simulink model "drone_control_definitivo"  (R2018a)
settings: Solver=FixedStepAuto  StartTime=0.0  StopTime=inf  FixedStep=sample_time  RelTol=1e-3
PostLoadFcn:
  | load('drone_buses.mat');
model workspace (MAT data in the model file):
  SL_ROS_VariableLengthArrays_MaxSizes.CommonInfo.ArrayTruncateAction = 'EmitWarning'
  SL_ROS_VariableLengthArrays_MaxSizes.MsgTypeMap = containers.Map
  SL_ROS_VariableLengthArrays_MaxSizes.MsgTypeMap.serialization.keys = {'sensor_msgs/Image'}
  SL_ROS_VariableLengthArrays_MaxSizes.MsgTypeMap.serialization.values{1}(1).PropertyName = 'Data'
  SL_ROS_VariableLengthArrays_MaxSizes.MsgTypeMap.serialization.values{1}(1).DataType = 'uint8'
  SL_ROS_VariableLengthArrays_MaxSizes.MsgTypeMap.serialization.values{1}(1).MaxLength = 230400
  SL_ROS_VariableLengthArrays_MaxSizes.MsgTypeMap.serialization.values{1}(2).PropertyName = 'Encoding'
  SL_ROS_VariableLengthArrays_MaxSizes.MsgTypeMap.serialization.values{1}(2).DataType = 'uint8'
  SL_ROS_VariableLengthArrays_MaxSizes.MsgTypeMap.serialization.values{1}(2).MaxLength = 128
  SL_ROS_VariableLengthArrays_MaxSizes.MsgTypeMap.serialization.uniformity = 0
  SL_ROS_VariableLengthArrays_MaxSizes.MsgTypeMap.serialization.keyType = 'char'
  SL_ROS_VariableLengthArrays_MaxSizes.MsgTypeMap.serialization.valueType = 'any'
  cmd_calibration = 0.4
  sample_time = 0.05
undefined symbols (not defined in the file or in its folder): Orientation, Position
libraries: robotlib x4, simulink_extras x2, simulink x2, aerolibanimutils x1
settings Model: Creator=rcasado  LastModifiedBy=dronechallenge
settings OptimizationCC: EnhancedBackFolding=on  PassReuseOutputArgsAs=Individual arguments  MaxStackSize=64  OptimizeBlockOrder=speed  DifferentSizesBufferReuse=on  OptimizationCustomize=off
settings DebuggingCC: ParameterTunabilityLossMsg=error  BusObjectLabelMismatch=none
settings HardwareCC: ProdBitPerPointer=32  ProdBitPerSizeT=32  ProdBitPerPtrDiffT=32  ProdLargestAtomicFloat=None  ProdIntDivRoundTo=Undefined  ProdEndianess=Unspecified  ProdWordSize=32  ProdHWDeviceType=Generic->Unspecified (assume 32-bit Generic)
settings SFSimCC: MATLABDynamicMemAlloc=off
settings RTWCC: SystemTargetFile=ert.tlc  HardwareBoard=Robot Operating System (ROS)  TLCOptions="-aInlineSetEventsForThisBaseRateFcn=TLC_FALSE -aSuppressMultiTaskScheduler=TLC_FALSE  -aRateBasedStepFcn=0"  TemplateMakefile=ert_default_tmf  GenerateReport=on  Toolchain=Catkin  IncludeHyperlinkInReport=on  LaunchReport=on  TargetLang=C++  GenerateTraceInfo=on  GenerateTraceReport=on  GenerateTraceReportSl=on  GenerateTraceReportSf=on  GenerateTraceReportEml=on
settings CodeAppCC: ForceParamTrailComments=on  IgnoreCustomStorageClasses=off  OperatorAnnotations=on  SimulinkDataObjDesc=on  SFDataObjDesc=on  InsertBlockDesc=on

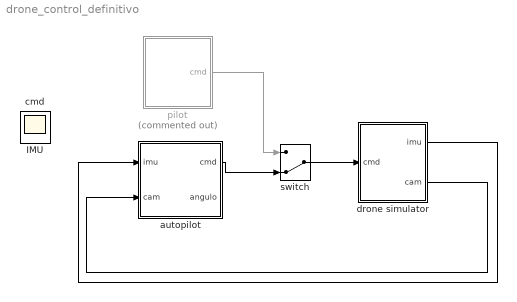
== system drone_control_definitivo ==
  autopilot : Stateflow chart  TreatAsAtomicUnit=on
  drone simulator : Subsystem
      mask Display:
      | patch([50 -50 -50 50], [40 40 -60 -60], [1 1 1])
      | 
      | patch([8 -8 -8 8], [6 6 -6 -6], [0.7 0.7 0.7])
      | 
      | patch([ 8  8  28  28], [2 0 0 2], [0.5 0.5 0.5])
      | patch([-8 -8 -28 -28], [2 0 0 2], [0.5 0.5 0.5])
      | 
      | patch([ 30  46  30  14], [6 5 4 5], [1 1 0])
      | patch([-30 -46 -30 -14], [6 5 4 5], [1 1 0])
      | 
      | patch([ 28  28  32  32], [4 -2 -2 4], [0 0 0])
      | patch([-28 -28 -32 -32], [4 -2 -2 4], [0 0 0])
      | 
      | patch([ 8  12  11  7], [-6 -18 -18 -6], [0 0 0])
      | patch([-8 -12 -11 -7], [-6 -18 -18 -6], [0 0 0])
  pilot : Subsystem  Commented=on
      mask Display:
      | patch([12 -2 -2 12], [12 12 -2 -2], [0.9 0.9 0.9])
      | 
      | % bola roja
      | patch([4 6 7 7 6 4 3 3], [6 6 7 9 10 10 9 7], [1 0 0])
      | 
      | % palo gris
      | patch([4 6 6 4], [3 3 6 6], [0.2 0.2 0.2])
      | 
      | % base negra
      | patch([1 9 10 10 9 1 0 0], [0 0 1 2 3 3 2 1], [0 0 0])
  switch : ManualSwitch  CurrentSetting=0
  IMU : Scope
  cmd : Scope
  wires:
  pilot/1(cmd) -> switch/1
  switch/1 -> drone simulator/1(cmd)
  autopilot/1(cmd) -> switch/2
  drone simulator/1(imu) -> autopilot/1(imu)
  drone simulator/2(cam) -> autopilot/2(cam)

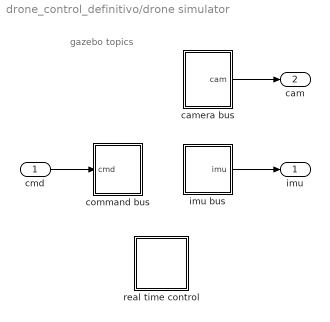
== system drone_control_definitivo/drone simulator ==
  note: gazebo
      | topics
  cmd : Inport
  camera bus : Subsystem
  command bus : Subsystem
  imu bus : Subsystem
  real time control : Subsystem
      mask Display: disp('realtime\ncontrol')
  imu : Outport
  cam : Outport  Port=2
  wires:
  imu bus/1(imu) -> imu/1
  cmd/1 -> command bus/1(cmd)
  camera bus/1(cam) -> cam/1

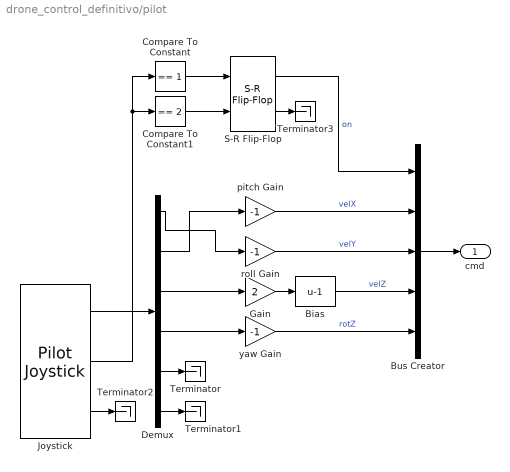
== system drone_control_definitivo/pilot ==
  Bias : Bias  Bias=-1
  Bus Creator : BusCreator  Inputs=5  OutDataTypeStr=Bus: bus_command  NonVirtualBus=on
      settings: InheritFromInputs=off
  Compare To Constant : simulink/Logic and Bit Operations/Compare To Constant  relop===  const=1  OutDataTypeStr=boolean
  Compare To Constant1 : simulink/Logic and Bit Operations/Compare To Constant  relop===  const=2  OutDataTypeStr=boolean
  Demux : Demux  Outputs=6
  Gain : Gain  Gain=2
  Joystick : aerolibanimutils/Pilot Joystick  JoystickID=Joystick1  OutputConfiguration=AllOutputs  SampleTime=sample_time
  S-R Flip-Flop : simulink_extras/Flip Flops/S-R Flip-Flop  initial_condition=0
  Terminator{,1..3} (4 alike) : Terminator
  pitch Gain : Gain  Gain=-1
  roll Gain : Gain  Gain=-1
  yaw Gain : Gain  Gain=-1
  cmd : Outport
  wires:
  Demux/4 -> yaw Gain/1
  Demux/3 -> Gain/1
  Demux/1 -> roll Gain/1
  Demux/2 -> pitch Gain/1
  Gain/1 -> Bias/1
  Bias/1 -> Bus Creator/4  "velZ"
  yaw Gain/1 -> Bus Creator/5  "rotZ"
  pitch Gain/1 -> Bus Creator/2  "velX"
  roll Gain/1 -> Bus Creator/3  "velY"
  S-R Flip-Flop/1 -> Bus Creator/1  "on"
  Bus Creator/1 -> cmd/1
  Joystick/1 -> Demux/1
  Demux/6 -> Terminator1/1
  Demux/5 -> Terminator/1
  Joystick/2 -> Compare To Constant/1, Compare To Constant1/1
  Joystick/3 -> Terminator2/1
  Compare To Constant/1 -> S-R Flip-Flop/1
  Compare To Constant1/1 -> S-R Flip-Flop/2
  S-R Flip-Flop/2 -> Terminator3/1

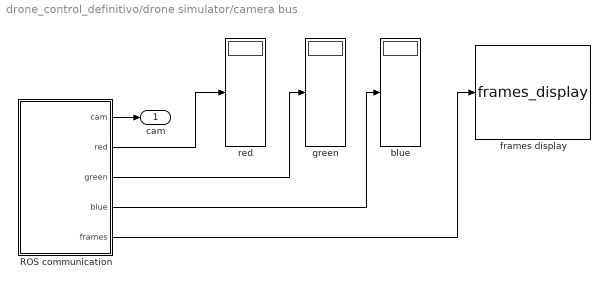
== system drone_control_definitivo/drone simulator/camera bus ==
  ROS communication : Subsystem
  blue : Display
  frames display : MATLABFcn  StartFcn=|  MATLABFcn=frames_display  OutputDimensions=0  Output1D=off
      | clear functions;
      | clc;
      mask Display:
      | patch([80 100 100 80], [60 60 80 80],[1 0 0])
      | 
      | patch([60 75 75 60], [20 20 30 30],[0 1 0])
      | 
      | patch([20 40 40 20], [40 40 50 50],[0 0 1])
  green : Display
  red : Display
  cam : Outport
  wires:
  ROS communication/2(red) -> red/1
  ROS communication/3(green) -> green/1
  ROS communication/4(blue) -> blue/1
  ROS communication/1(cam) -> cam/1
  ROS communication/5(frames) -> frames display/1

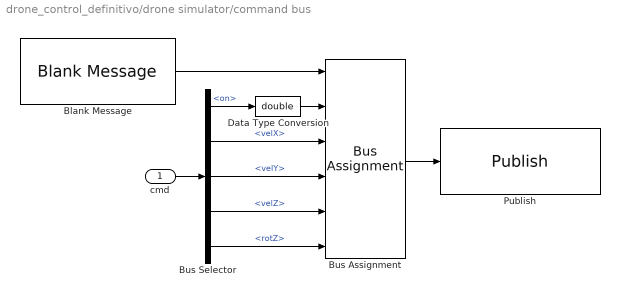
== system drone_control_definitivo/drone simulator/command bus ==
  cmd : Inport
  Blank Message : robotlib/Blank Message  SourceLibraryInfo=This block requires Robotics System Toolbox  messageType=geometry_msgs/Pose  SampleTime=sample_time
      settings: SourceProductBaseCode=RO
  Bus Assignment : BusAssignment  AssignedSignals=Position.X,Orientation.X,Orientation.Y,Orientation.Z,Orientation.W
  Bus Selector : BusSelector  OutputSignals=on,velX,velY,velZ,rotZ
  Data Type Conversion : DataTypeConversion  OutDataTypeStr=double
  Publish : robotlib/Publish  SourceLibraryInfo=This block requires Robotics System Toolbox  topicSource=Select from ROS network  topic=/quadcopter/bus_command  messageType=geometry_msgs/Pose  messageQueueLength=105
      settings: SourceProductBaseCode=RO
  wires:
  Bus Assignment/1 -> Publish/1
  cmd/1 -> Bus Selector/1
  Blank Message/1 -> Bus Assignment/1
  Bus Selector/4 -> Bus Assignment/5  "<velZ>"
  Bus Selector/3 -> Bus Assignment/4  "<velY>"
  Bus Selector/2 -> Bus Assignment/3  "<velX>"
  Bus Selector/1 -> Data Type Conversion/1  "<on>"
  Bus Selector/5 -> Bus Assignment/6  "<rotZ>"
  Data Type Conversion/1 -> Bus Assignment/2

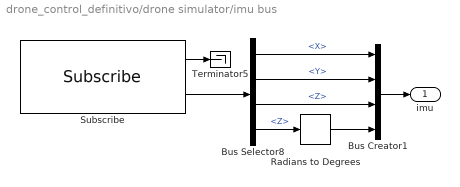
== system drone_control_definitivo/drone simulator/imu bus ==
  Bus Creator1 : BusCreator  Inputs=4  OutDataTypeStr=Bus: bus_IMU  NonVirtualBus=on
      settings: InheritFromInputs=off
  Bus Selector8 : BusSelector  DialogController=Simulink.DDGSource_BusSelector  OutputSignals=Pose.Position.X,Pose.Position.Y,Pose.Position.Z,Pose.Orientation.Z
  Radians to Degrees : simulink_extras/Transformations/Radians to Degrees
  Subscribe : robotlib/Subscribe  SourceLibraryInfo=This block requires Robotics System Toolbox  topicSource=Select from ROS network  topic=/quadcopter/odometry  messageType=gazebo_msgs/ModelState  sampleTime=sample_time  messageQueueLength=51
      settings: SourceProductBaseCode=RO
  Terminator5 : Terminator
  imu : Outport
  wires:
  Subscribe/1 -> Terminator5/1
  Bus Selector8/4 -> Radians to Degrees/1  "<Z>"
  Bus Selector8/2 -> Bus Creator1/2  "<Y>"
  Bus Selector8/3 -> Bus Creator1/3  "<Z>"
  Bus Selector8/1 -> Bus Creator1/1  "<X>"
  Bus Creator1/1 -> imu/1
  Radians to Degrees/1 -> Bus Creator1/4
  Subscribe/2 -> Bus Selector8/1

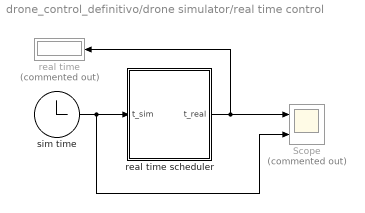
== system drone_control_definitivo/drone simulator/real time control ==
  Scope : Scope  Commented=on  NumInputPorts=2
  real time : Display  Commented=on
      settings: Format=bank
  real time scheduler : MATLAB Function  TreatAsAtomicUnit=on
  sim time : Clock
  wires:
  real time scheduler/1(t_real) -> real time/1, Scope/1
  sim time/1 -> real time scheduler/1(t_sim), Scope/2

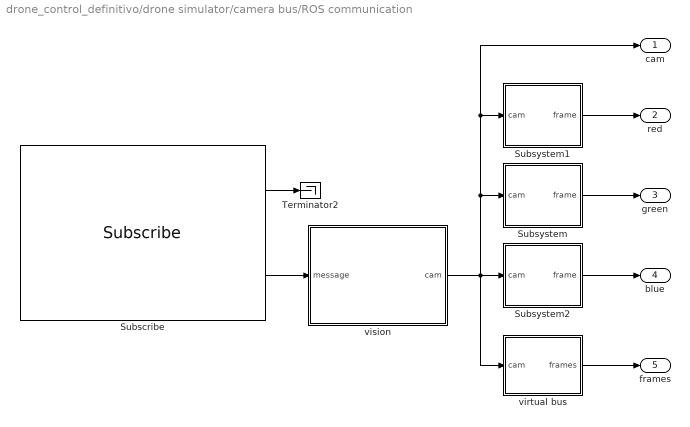
== system drone_control_definitivo/drone simulator/camera bus/ROS communication ==
  Subscribe : robotlib/Subscribe  SourceLibraryInfo=This block requires Robotics System Toolbox  topicSource=Select from ROS network  topic=/quadcopter/onboard_camera/image_raw  messageType=sensor_msgs/Image  sampleTime=sample_time  messageQueueLength=51
      settings: SourceProductBaseCode=RO
  Subsystem : Subsystem
  Subsystem1 : Subsystem
  Subsystem2 : Subsystem
  Terminator2 : Terminator
  virtual bus : Subsystem
  vision : MATLAB Function  TreatAsAtomicUnit=on
  cam : Outport
  red : Outport  Port=2
  green : Outport  Port=3
  blue : Outport  Port=4
  frames : Outport  Port=5
  wires:
  Subsystem/1(frame) -> green/1
  Subsystem1/1(frame) -> red/1
  Subsystem2/1(frame) -> blue/1
  virtual bus/1(frames) -> frames/1
  vision/1(cam) -> cam/1, Subsystem1/1(cam), Subsystem/1(cam), virtual bus/1(cam), Subsystem2/1(cam)
  Subscribe/2 -> vision/1(message)
  Subscribe/1 -> Terminator2/1

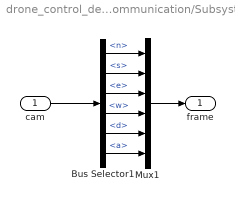
== system drone_control_definitivo/drone simulator/camera bus/ROS communication/Subsystem ==
  cam : Inport
  Bus Selector1 : BusSelector  OutputSignals=green.n,green.s,green.e,green.w,green.d,green.a
  Mux1 : Mux  Inputs=6
  frame : Outport
  wires:
  Bus Selector1/3 -> Mux1/3  "<e>"
  Bus Selector1/6 -> Mux1/6  "<a>"
  Bus Selector1/5 -> Mux1/5  "<d>"
  Bus Selector1/4 -> Mux1/4  "<w>"
  cam/1 -> Bus Selector1/1
  Bus Selector1/1 -> Mux1/1  "<n>"
  Mux1/1 -> frame/1
  Bus Selector1/2 -> Mux1/2  "<s>"

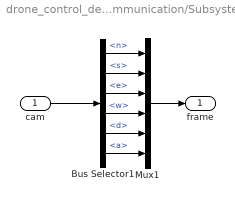
== system drone_control_definitivo/drone simulator/camera bus/ROS communication/Subsystem1 ==
  cam : Inport
  Bus Selector1 : BusSelector  OutputSignals=red.n,red.s,red.e,red.w,red.d,red.a
  Mux1 : Mux  Inputs=6
  frame : Outport
  wires:
  Bus Selector1/3 -> Mux1/3  "<e>"
  Bus Selector1/6 -> Mux1/6  "<a>"
  Bus Selector1/5 -> Mux1/5  "<d>"
  Bus Selector1/4 -> Mux1/4  "<w>"
  cam/1 -> Bus Selector1/1
  Bus Selector1/1 -> Mux1/1  "<n>"
  Mux1/1 -> frame/1
  Bus Selector1/2 -> Mux1/2  "<s>"

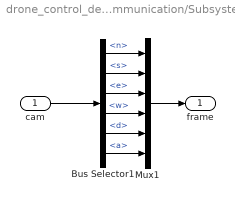
== system drone_control_definitivo/drone simulator/camera bus/ROS communication/Subsystem2 ==
  cam : Inport
  Bus Selector1 : BusSelector  OutputSignals=blue.n,blue.s,blue.e,blue.w,blue.d,blue.a
  Mux1 : Mux  Inputs=6
  frame : Outport
  wires:
  Bus Selector1/3 -> Mux1/3  "<e>"
  Bus Selector1/6 -> Mux1/6  "<a>"
  Bus Selector1/5 -> Mux1/5  "<d>"
  Bus Selector1/4 -> Mux1/4  "<w>"
  cam/1 -> Bus Selector1/1
  Bus Selector1/1 -> Mux1/1  "<n>"
  Mux1/1 -> frame/1
  Bus Selector1/2 -> Mux1/2  "<s>"

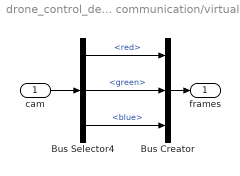
== system drone_control_definitivo/drone simulator/camera bus/ROS communication/virtual bus ==
  cam : Inport
  Bus Creator : BusCreator  Inputs=3  OutDataTypeStr=Bus: bus_camera
      settings: InheritFromInputs=off
  Bus Selector4 : BusSelector  OutputSignals=red,green,blue
  frames : Outport
  wires:
  Bus Selector4/1 -> Bus Creator/1  "<red>"
  Bus Selector4/3 -> Bus Creator/3  "<blue>"
  Bus Selector4/2 -> Bus Creator/2  "<green>"
  cam/1 -> Bus Selector4/1
  Bus Creator/1 -> frames/1

== matlab function drone_control_definitivo/drone simulator/real time control/real time scheduler ==
  data: t_sim input; t_real output
function t_real = fcn(t_sim)
%#codegen

coder.extrinsic('tic');
coder.extrinsic('toc');

persistent t0;
if isempty(t0)
    t0 = tic;
    t_real = 0;
end

t_real = toc(t0);

t_dif = t_sim - t_real;
if t_dif > 0
%    disp(t_dif)
    pause(t_dif);
end

t_real = toc(t0);
%disp(t_real)

== stateflow chart drone_control_definitivo/autopilot ==
  settings: updateMethod=DISCRETE  sampleTime=sample_time  executeAtInitialization=1
  state nav1 [parallel] [commented out]
    state inicio [commented out]
      entry:
      cmd.on=true;
    state AscenderA3m [commented out]
      entry:
      alturaFinal=3.00;
      during:
      velocidadZ=alturaFinal-imu.posZ;
      cmd.velZ=velocidadZ;
    state Suspendido [commented out]
      entry:
      cmd.velZ=0.00;
    state DescenderA2m [commented out]
      entry:
      alturaFinal=2.00;
      during:
      velocidadZ = alturaFinal-imu.posZ;
      cmd.velZ=velocidadZ;
    state Suspendido1 [commented out]
      entry:
      cmd.velZ=0.00;
    (default) -> nav1.inicio [commented out]
    nav1.inicio -> AscenderA3m [commented out]
    Suspendido1 -> AscenderA3m [commented out] : after(3,sec)
    AscenderA3m -> Suspendido [commented out] : [abs(alturaFinal - imu.posZ) < 0.01]
    Suspendido -> DescenderA2m [commented out] : after(3,sec)
    DescenderA2m -> Suspendido1 [commented out] : [abs(alturaFinal - imu.posZ) < 0.01]
  state nav2 [parallel] [commented out]
    state inicio [commented out]
      entry:
      cmd.on= true;
    state PosicionInicial [commented out]
      entry:
      posXInit = imu.posX;
      posYInit = imu.posY;
      posZInit = imu.posZ;
    state Ir [commented out]
      entry:
      dist = inf;
      during:
      dist = FlyTo(3,2,1);
    state Posicionar [commented out]
      entry:
      during:
      Look2Frame('red');
    (default) -> nav2.inicio [commented out]
    nav2.inicio -> PosicionInicial [commented out]
    PosicionInicial -> Ir [commented out]
    Posicionar -> Ir [commented out] : [cam.red.d < 0.45]
  state sobrevolar [parallel] [commented out]
    state despegar [commented out]
      entry:
      Hover
    state mantener [commented out]
      Hover
    state al_centro [commented out]
      entry:
      dist = inf;
      during:
      dist = FlyTo(0,0,1);
    (default) -> despegar [commented out]
    despegar -> al_centro [commented out]
    al_centro -> mantener [commented out] : [dist < 0.2]
  state main [parallel]
    settings: executionOrder=1
    state Despegar
      state Arrancar
        entry:
        cmd.on = true;
      state guardar_posInicial
        entry:
        posXInit = imu.posX;
        posYInit = imu.posY;
        posZInit = imu.posZ;
      state Fin
      (default) -> Arrancar
      Arrancar -> guardar_posInicial
      guardar_posInicial -> Fin
    state Atraviesa_marco_azul
      state voy_al_centro
        entry:
      state loveo
        entry:
        Hover();
        during:
        Look2Frame('blue');
        EsquivarObstaculo('blue');
        cmd.velX = min((cam.blue.d-0.4)/2,1);
      state excepcion_bm1
        entry:
        Hover
        cmd.rotZ = 1;
        cmd.velZ = 0.2;
        during:
        FlyTo2D(0,0);
      state buscar_marco
        entry:
        Hover
        dist = inf;
        cmd.rotZ = 1;
        during:
        dist =FlyTo(0,0,1);
      state cerca
        entry:
        Hover
        initA = cam.blue.a;
      state exception_bm2
        entry:
        Hover
        cmd.rotZ = 1;
        during:
        cmd.velZ = -0.2;
        FlyTo2D(-2,-2);
      state desplaz_izquierda
        entry:
        during:
        Look2Frame('blue');
        RotarMarco('blue',0);
      state desplaz_derecha
        entry:
        during:
        Look2Frame('blue');
        RotarMarco('blue',1);
      state cruza
        entry:
        Hover
        altura = imu.posZ;
        during:
        Atravesar(altura);
      (default) -> main.Atraviesa_marco_azul.voy_al_centro
      main.Atraviesa_marco_azul.loveo -> main.Atraviesa_marco_azul.voy_al_centro [order 2] : [cam.blue.d == inf]
      main.Atraviesa_marco_azul.voy_al_centro -> main.Atraviesa_marco_azul.loveo [order 1] : [cam.blue.d ~= inf ]
      main.Atraviesa_marco_azul.voy_al_centro -> main.Atraviesa_marco_azul.buscar_marco [order 2] : [cam.red.d == inf]
      main.Atraviesa_marco_azul.buscar_marco -> main.Atraviesa_marco_azul.loveo [order 1] : [cam.blue.d ~= inf]
      main.Atraviesa_marco_azul.loveo -> main.Atraviesa_marco_azul.cerca [order 1] : [cam.blue.d < 0.45]
      main.Atraviesa_marco_azul.buscar_marco -> main.Atraviesa_marco_azul.excepcion_bm1 [order 2] : [after(5,sec)]
      main.Atraviesa_marco_azul.excepcion_bm1 -> main.Atraviesa_marco_azul.exception_bm2 [order 2] : [after(13,sec)]
      main.Atraviesa_marco_azul.excepcion_bm1 -> main.Atraviesa_marco_azul.buscar_marco [order 1] : [cam.blue.d ~= inf]
      main.Atraviesa_marco_azul.exception_bm2 -> main.Atraviesa_marco_azul.excepcion_bm1 [order 2] : [after(13,sec)]
      main.Atraviesa_marco_azul.cerca -> main.Atraviesa_marco_azul.desplaz_izquierda
      main.Atraviesa_marco_azul.exception_bm2 -> main.Atraviesa_marco_azul.buscar_marco [order 1] : [cam.blue.d ~= inf]
      main.Atraviesa_marco_azul.desplaz_izquierda -> main.Atraviesa_marco_azul.desplaz_derecha [order 2] : [initA < cam.blue.a]
      main.Atraviesa_marco_azul.desplaz_izquierda -> main.Atraviesa_marco_azul.cruza [order 1] : [cam.blue.a < 10]
      main.Atraviesa_marco_azul.desplaz_derecha -> main.Atraviesa_marco_azul.cruza : [cam.blue.a < 10]
    state Atraviesa_marco_rojo
      state voy_al_centro
        entry:
      state loveo
        entry:
        Hover();
        during:
        Look2Frame('red');
        EsquivarObstaculo('red');
        cmd.velX = min((cam.red.d-0.4)/2,1);
      state excepcion_bm1
        entry:
        Hover
        cmd.rotZ = 1;
        cmd.velZ = 0.2;
        during:
        FlyTo2D(0,0);
      state buscar_marco
        entry:
        Hover
        dist = inf;
        cmd.rotZ = 1;
        during:
        dist =FlyTo(0,0,1);
      state cerca
        entry:
        Hover
      state exception_bm2
        entry:
        Hover
        cmd.rotZ = 1;
        during:
        cmd.velZ = -0.2;
        FlyTo2D(-2,-2);
      state desplaz_izquierda
        entry:
        during:
        Look2Frame('red');
        RotarMarco('red',0);
      state desplaz_derecha
        entry:
        during:
        Look2Frame('red');
        RotarMarco('red',1);
      state cruza
        entry:
        Hover
        altura = imu.posZ;
        during:
        Atravesar(altura);
      (default) -> main.Atraviesa_marco_rojo.voy_al_centro
      main.Atraviesa_marco_rojo.loveo -> main.Atraviesa_marco_rojo.voy_al_centro [order 2] : [cam.red.d == inf]
      main.Atraviesa_marco_rojo.voy_al_centro -> main.Atraviesa_marco_rojo.buscar_marco [order 2] : [cam.red.d == inf]
      main.Atraviesa_marco_rojo.voy_al_centro -> main.Atraviesa_marco_rojo.loveo [order 1] : [cam.red.d ~= inf ]
      main.Atraviesa_marco_rojo.buscar_marco -> main.Atraviesa_marco_rojo.loveo [order 1] : [cam.red.d ~= inf]
      main.Atraviesa_marco_rojo.loveo -> main.Atraviesa_marco_rojo.cerca [order 1] : [cam.red.d < 0.45]
      main.Atraviesa_marco_rojo.buscar_marco -> main.Atraviesa_marco_rojo.excepcion_bm1 [order 2] : [after(5,sec)]
      main.Atraviesa_marco_rojo.excepcion_bm1 -> main.Atraviesa_marco_rojo.exception_bm2 [order 2] : [after(13,sec)]
      main.Atraviesa_marco_rojo.excepcion_bm1 -> main.Atraviesa_marco_rojo.buscar_marco [order 1] : [cam.red.d ~= inf]
      main.Atraviesa_marco_rojo.exception_bm2 -> main.Atraviesa_marco_rojo.excepcion_bm1 [order 2] : [after(13,sec)]
      main.Atraviesa_marco_rojo.cerca -> main.Atraviesa_marco_rojo.desplaz_izquierda : after(0.2,sec){initA = cam.red.a}
      main.Atraviesa_marco_rojo.exception_bm2 -> main.Atraviesa_marco_rojo.buscar_marco [order 1] : [cam.red.d ~= inf]
      main.Atraviesa_marco_rojo.desplaz_izquierda -> main.Atraviesa_marco_rojo.desplaz_derecha [order 2] : [initA < cam.red.a]
      main.Atraviesa_marco_rojo.desplaz_izquierda -> main.Atraviesa_marco_rojo.cruza [order 1] : [cam.red.a < 10]
      main.Atraviesa_marco_rojo.desplaz_derecha -> main.Atraviesa_marco_rojo.cruza : [cam.red.a < 10]
    state Atraviesa_marco_verde
      state voy_al_centro
        entry:
      state loveo
        entry:
        Hover();
        during:
        Look2Frame('green');
        EsquivarObstaculo('green');
        cmd.velX = min((cam.green.d-0.4)/2,1);
      state excepcion_bm1
        entry:
        Hover
        cmd.rotZ = 1;
        cmd.velZ = 0.2;
        during:
        FlyTo2D(0,0);
      state buscar_marco
        entry:
        Hover
        dist = inf;
        cmd.rotZ = 1;
        during:
        dist =FlyTo(0,0,1);
      state cerca
        entry:
        Hover
        initA = (cam.green.a+5)
      state exception_bm2
        entry:
        Hover
        cmd.rotZ = 1;
        during:
        cmd.velZ = -0.2;
        FlyTo2D(-2,-2);
      state desplaz_izquierda
        entry:
        during:
        Look2Frame('green');
        RotarMarco('green',0);
      state desplaz_derecha
        entry:
        during:
        Look2Frame('green');
        RotarMarco('green',1);
      state cruza
        entry:
        Hover
        altura = imu.posZ;
        during:
        Atravesar(altura);
      (default) -> main.Atraviesa_marco_verde.voy_al_centro
      main.Atraviesa_marco_verde.loveo -> main.Atraviesa_marco_verde.voy_al_centro [order 2] : [cam.green.d == inf]
      main.Atraviesa_marco_verde.voy_al_centro -> main.Atraviesa_marco_verde.buscar_marco [order 2] : [cam.green.d == inf]
      main.Atraviesa_marco_verde.voy_al_centro -> main.Atraviesa_marco_verde.loveo [order 1] : [cam.green.d ~= inf ]
      main.Atraviesa_marco_verde.buscar_marco -> main.Atraviesa_marco_verde.loveo [order 1] : [cam.green.d ~= inf]
      main.Atraviesa_marco_verde.loveo -> main.Atraviesa_marco_verde.cerca [order 1] : [cam.green.d < 0.45]
      main.Atraviesa_marco_verde.buscar_marco -> main.Atraviesa_marco_verde.excepcion_bm1 [order 2] : [after(5,sec)]
      main.Atraviesa_marco_verde.excepcion_bm1 -> main.Atraviesa_marco_verde.exception_bm2 [order 2] : [after(13,sec)]
      main.Atraviesa_marco_verde.excepcion_bm1 -> main.Atraviesa_marco_verde.buscar_marco [order 1] : [cam.green.d ~= inf]
      main.Atraviesa_marco_verde.exception_bm2 -> main.Atraviesa_marco_verde.excepcion_bm1 [order 2] : [after(13,sec)]
      main.Atraviesa_marco_verde.cerca -> main.Atraviesa_marco_verde.desplaz_izquierda
      main.Atraviesa_marco_verde.exception_bm2 -> main.Atraviesa_marco_verde.buscar_marco [order 1] : [cam.green.d ~= inf]
      main.Atraviesa_marco_verde.desplaz_izquierda -> main.Atraviesa_marco_verde.desplaz_derecha [order 2] : [initA < cam.green.a]
      main.Atraviesa_marco_verde.desplaz_izquierda -> main.Atraviesa_marco_verde.cruza [order 1] : [cam.green.a < 10]
      main.Atraviesa_marco_verde.desplaz_derecha -> main.Atraviesa_marco_verde.cruza : [cam.green.a < 10]
    state Aterrizar
      state Volver_a_base
        entry:
        Hover
        dist = inf;
        during:
        dist = FlyTo(posXInit, posYInit,(posZInit+0.1));
      state Apagar
        entry:
        Hover
        cmd.on = false;
      (default) -> Volver_a_base
      Volver_a_base -> Apagar : [dist < 0.1]
    (default) -> Despegar
    main.Atraviesa_marco_rojo.cruza -> Atraviesa_marco_verde : [after(1.5,sec)]
    main.Atraviesa_marco_verde.cruza -> Atraviesa_marco_azul : [after(1.5,sec)]
    main.Atraviesa_marco_azul.cruza -> Aterrizar : [after(1.5,sec)]
    Fin -> Atraviesa_marco_rojo
  data: X function_input; Y function_input; Z function_input; d3D function_output; id function_input; X function_input; Y function_input; d2D function_output; id function_input; Z function_input; color function_input; ang function_output; direccion function_input; imu input Bus: bus_IMU size=1; cmd output Bus: bus_command size=1 =0; cam input Bus: bus_camera size=1; alturaFinal local; velocidadZ local; posXInit local double; posYInit local double; posZInit local double; dist local; init local; initA local; marco local; posXMarco local; altura local; angulo output
  function d3D = FlyTo(X,Y,Z):
    | function d3D = FlyTo(X,Y,Z)
    | 
    | %distancia a bojetivo
    | %expresada en ejes del suelo
    | dxs = X - imu.posX;
    | dys = Y - imu.posY;
    | dzs = Z - imu.posZ;
    | 
    | %Distancia a objetivo
    | d3D = norm([dxs dys dzs]);
    | 
    | %distacia a objetivo sobre el plano
    | d2D = norm([dxs dys]);
    | 
    | %angulo enrte el morro del drone y el objetivo
    | angulo = atan2d(dys, dxs) - imu.rumbo;
    | 
    | %distancia a objetivo sobre el plano
    | %expresada en ejes del drone
    | dx = d2D*cosd(angulo);
    | dy = d2D*sind(angulo);
    | 
    | %velocidad sobre el plano (reducida a la mitad)
    | %expresada en ejes del drone
    | vel2D = [dx dy] / 2;
    | if norm(vel2D) > 1
    |     vel2D = vel2D / norm(vel2D);
    | end
    | 
    | %velocidad vertical
    | velZ = min(dzs/2, 1);
    | 
    | cmd.velX = vel2D(1);
    | cmd.velY = vel2D(2);
    | cmd.velZ = velZ;
  function EsquivarObstaculo(id):
    | function EsquivarObstaculo(id)
    | 
    | switch id
    |     case 'red'
    |         obs1 = cam.green;
    |         obs2 = cam.blue;
    |     case 'green'
    |         obs1 = cam.red;
    |         obs2 = cam.blue;
    |     case 'blue'
    |         obs1 = cam.red;
    |         obs2 = cam.green;
    | end
    | 
    | 
    | if((abs(obs1.w) + obs1.e) < 100)
    |     cmd.velY = 0.5;
    | else
    |     if((abs(obs2.w) + obs2.e) < 100)
    |         cmd.velY = 0.5;
    |     else
    |         cmd.velY = 0;
    |     end
    | end
  function d2D = FlyTo2D(X, Y):
    | function d2D = FlyTo2D(X, Y)
    | 
    | %distancia a bojetivo
    | %expresada en ejes del suelo
    | dxs = X - imu.posX;
    | dys = Y - imu.posY;
    | 
    | 
    | %distacia a objetivo sobre el plano
    | d2D = norm([dxs dys]);
    | 
    | %angulo enrte el morro del drone y el objetivo
    | angulo = atan2d(dys, dxs) - imu.rumbo;
    | 
    | %distancia a objetivo sobre el plano
    | %expresada en ejes del drone
    | dx = d2D*cosd(angulo);
    | dy = d2D*sind(angulo);
    | 
    | %velocidad sobre el plano (reducida a la mitad)
    | %expresada en ejes del drone
    | vel2D = [dx dy] / 2;
    | if norm(vel2D) > 1
    |     vel2D = vel2D / norm(vel2D);
    | end
    | 
    | cmd.velX = vel2D(1);
    | cmd.velY = vel2D(2);
  function Look2Frame(id):
    | function Look2Frame(id)
    | 
    | switch id
    |     case 'red'
    |         fr = cam.red;
    |     case 'green'
    |         fr = cam.green;
    |     case 'blue'
    |         fr = cam.blue;
    | end
    | cmd.velX = (fr.d-0.3)/8;
    | if (fr.d ~= inf)
    |     HorCenter = (fr.e + fr.w) / 2;
    |     cmd.rotZ = - HorCenter / 80;
    |     VerCenter = (fr.n + fr.s) / 2;
    |     cmd.velZ = VerCenter/120;
    | end
  function Hover:
    | function Hover
    | cmd.on = true;
    |  cmd.velX = 0;
    |  cmd.velY = 0;
    |  cmd.velZ = 0;
    |  cmd.rotZ = 0;
  function Atravesar(Z):
    | function Atravesar(Z)
    | dz = Z - imu.posZ;
    | 
    | %velocidad vertical
    | velZ = min(dz/2, 1);
    | 
    | %velocidades
    | cmd.velX = 1;
    | cmd.velZ = velZ;
  function ang = RotarMarco(color, direccion):
    | function ang = RotarMarco(color, direccion)
    | switch color
    |     case 'red'
    |         fr = cam.red;
    |     case 'green'
    |         fr = cam.green;
    |     case 'blue'
    |         fr = cam.blue;
    | end
    | 
    | if(direccion == 1)%derecha
    |     velY = (fr.a/200);
    |     cmd.velY = -velY;
    |     
    | else
    |     velY = (fr.a/200);
    |     cmd.velY = velY;%izquierda
    | end

== matlab function drone_control_definitivo/drone simulator/camera bus/ROS communication/vision ==
  data: message input; cam output Bus: bus_camera
function cam = fcn(message)

% leemos la imagen
width  = message.Width;
height = message.Height;
img    = message.Data;

% establecemos los valores umbrales de deteccion de color
th1 = 50;         % umbral entre color primario y secundarios
th2 = 20;         % umbral entre colores secundarios

% marco rojo
frame_red.d = +inf;        % distancia estimada
frame_red.a = +inf;        % angulo de entrada estimado
frame_red.n = +inf;        % lado norte
frame_red.s = -inf;        % lado sur
frame_red.e = -inf;        % lado este
frame_red.w = +inf;        % lado oeste

% marco verde
frame_green = frame_red;      
% marco azul
frame_blue = frame_red; 


% deteccion de rectangulos conteniendo los pixeles de cada marco
i = 1;
for row = 1:height %240
for col = 1:width  %320

    r = double(img(i));  i=i+1;
    g = double(img(i));  i=i+1;
    b = double(img(i));  i=i+1;
    
    if(abs(g-b) < th2) && ((r-g) > th1)        %rojo
        if(frame_red.n > row) 
           frame_red.n = double(row);
        end
        if(frame_red.s < row) 
           frame_red.s = double(row);
        end
        if(frame_red.e < col) 
           frame_red.e = double(col);
        end
        if(frame_red.w > col) 
           frame_red.w = double(col);
        end
    elseif(abs(b-r) < th2) && ((g-b) > th1)    %verde
        if(frame_green.n > row) 
           frame_green.n = double(row);
        end
        if(frame_green.s < row) 
           frame_green.s = double(row);
        end
        if(frame_green.e < col) 
           frame_green.e = double(col);
        end
        if(frame_green.w > col) 
           frame_green.w = double(col);
        end
    elseif(abs(r-g) < th2) && ((b-r) > th1)    %azul
        if(frame_blue.n > row) 
           frame_blue.n = double(row);
        end
        if(frame_blue.s < row) 
           frame_blue.s = double(row);
        end
        if(frame_blue.e < col) 
           frame_blue.e = double(col);
        end
        if(frame_blue.w > col) 
           frame_blue.w = double(col);
        end
    end
    
end
end

% Cambio del sistema de coordenadas de la imagen
frame_red.n   = 120 - frame_red.n;
frame_red.s   = 120 - frame_red.s;
frame_red.e   = frame_red.e - 161;
frame_red.w   = frame_red.w - 161;

frame_green.n = 120 - frame_green.n;
frame_green.s = 120 - frame_green.s;
frame_green.e = frame_green.e - 161;
frame_green.w = frame_green.w - 161;

frame_blue.n  = 120 - frame_blue.n;
frame_blue.s  = 120 - frame_blue.s;
frame_blue.e  = frame_blue.e - 161;
frame_blue.w  = frame_blue.w - 161;


%% Analisis de posicion (distancia, y angulos de deriva/entrada)

d2 = 160^2;    % 160^2 pixeles
L  = 0.23;       % alto de marco
A  = 0.43;       % ancho del marco

if frame_red.n > -inf && frame_red.n < 119 && frame_red.s > -120
    l = frame_red.n - frame_red.s;
    h = frame_red.s + l/2;
    frame_red.d = L/l * sqrt(d2 + h^2);
    ap = frame_red.e - frame_red.w;
    a = max(A/L * l,ap);
    frame_red.a = acosd(ap/a);
end

if frame_green.n > -inf && frame_green.n < 119 && frame_green.s > -120
    l = frame_green.n - frame_green.s;
    h = frame_green.s + l/2;
    frame_green.d = L/l * sqrt(d2 + h^2);
    ap = frame_green.e - frame_green.w;
    a = max(A/L * l,ap);
    frame_green.a = acosd(ap/a);
end

if frame_blue.n > -inf && frame_blue.n < 119 && frame_blue.s > -120
    l = frame_blue.n - frame_blue.s;
    h = frame_blue.s + l/2;
    frame_blue.d = L/l * sqrt(d2 + h^2);
    ap = frame_blue.e - frame_blue.w;
    a = max(A/L * l,ap);
    frame_blue.a = acosd(ap/a);
end




%% Enviamos informacion por el topic
cam.red = frame_red;
cam.green = frame_green;
cam.blue = frame_blue;
